simulink model "decision"  (R2015a)
settings: Solver=ode45  StartTime=0.0  StopTime=10.0  RelTol=1e-3
settings Model: Creator=Sneha More  LastModifiedBy=Sneha More

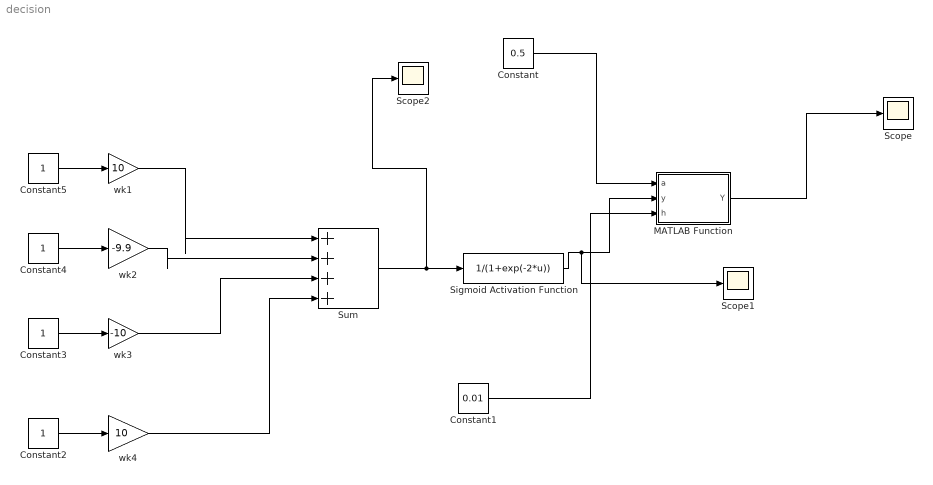
== system decision ==
  Constant : Constant  Value=0.5
  Constant1 : Constant  Value=0.01
  Constant{2..5} (4 alike) : Constant
  MATLAB Function : MATLAB Function  TreatAsAtomicUnit=on
  Scope : Scope
  Scope1 : Scope
  Scope2 : Scope
      settings: SaveName=ScopeData2
  Sigmoid Activation Function : Fcn  Expr=1/(1+exp(-2*u))
  Sum : Sum  Inputs=|++++
  wk1 : Gain  Gain=10
  wk2 : Gain  Gain=-9.9
  wk3 : Gain  Gain=-10
  wk4 : Gain  Gain=10
  wires:
  Constant5/1 -> wk1/1
  Constant4/1 -> wk2/1
  Constant3/1 -> wk3/1
  Constant2/1 -> wk4/1
  wk1/1 -> Sum/1
  wk2/1 -> Sum/2
  wk3/1 -> Sum/3
  wk4/1 -> Sum/4
  Sum/1 -> Scope2/1, Sigmoid Activation Function/1
  Sigmoid Activation Function/1 -> Scope1/1, MATLAB Function/2(y)
  MATLAB Function/1(Y) -> Scope/1
  Constant/1 -> MATLAB Function/1(a)
  Constant1/1 -> MATLAB Function/3(h)

== matlab function decision/MATLAB Function ==
  data: a input; y input; h input; Y output
function Y = fgl_deriv( a, y, h )
%#codegen

 n  = numel(y);
    J  = 0:(n-1);
    G1 = gamma( J+1 );
    G2 = gamma( a+1-J );
    s  = (-1) .^ J;

    M  = tril( ones(n) );
    R  = toeplitz( y(:)' );
    T  = meshgrid( (gamma(a+1)/(h^a)) * s ./ (G1.*G2) );
    Y  = reshape(sum( R .* M .* T, 2 ), size(y));
    
    
end
